simulink model "Quadrotor"  (R2017a)
settings: Solver=FixedStepAuto  StartTime=0.0  StopTime=12  FixedStep=0.001  RelTol=1e-3  EnableMultiTasking=on
values from neighbouring files (symbols this model uses):
  dU0 = 0*ones(Usize,1)    [go.m]
  U0 = 0*ones(Usize,1)    [go.m]
settings Model: Creator=stajeddi  LastModifiedBy=stajeddi
settings DataIOCC: LimitDataPoints=on
settings OptimizationCC: LifeSpan=inf
settings DebuggingCC: AllowSymbolicDim=off  SFUnexpectedBacktrackingDiag=warning  SFNoUnconditionalDefaultTransitionDiag=warning  SFExecutionAtInitializationDiag=none
settings ModelReferenceCC: PropagateSignalLabelsOutOfModel=off
settings GRTTargetCC: TargetLangStandard=C89/C90 (ANSI)
settings ConfigComp: CovMetricSettings=dw  CovHtmlReporting=on  CovSaveCumulativeToWorkspaceVar=on  CovSaveSingleToWorkspaceVar=on  CovExternalEMLEnable=off

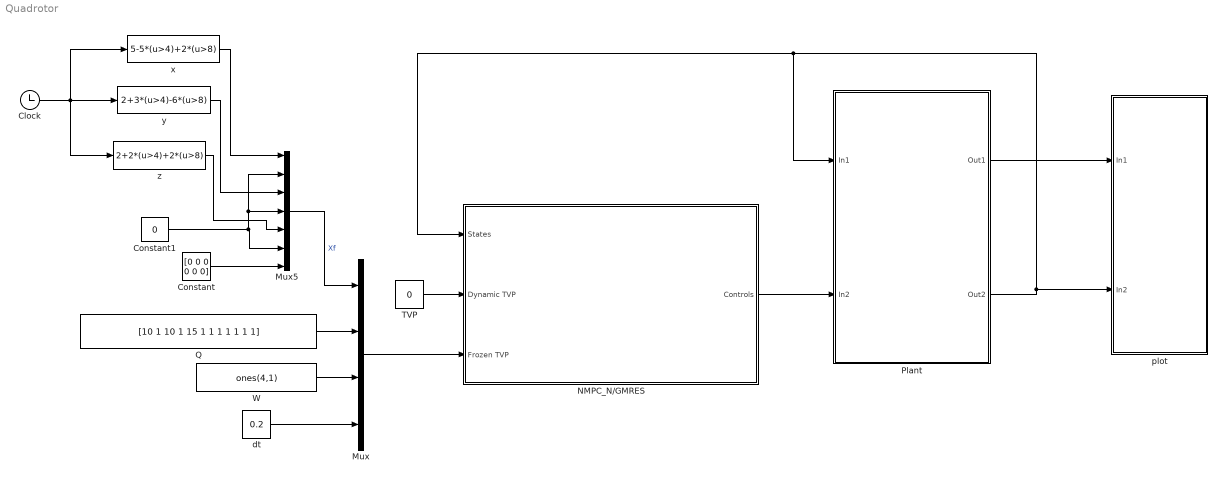
== system Quadrotor ==
  Clock : Clock
  Constant : Constant  Value=[0 0 0 0 0 0]
  Constant1 : Constant  Value=0
  Mux : Mux
  Mux5 : Mux  Inputs=7
  NMPC_N/GMRES : Subsystem
  Plant : Subsystem
  Q : Constant  Value=[10 1 10 1 15 1 1 1 1 1 1 1]
  TVP : Constant  Value=0
  W : Constant  Value=ones(4,1)
  dt : Constant  Value=0.2
  plot : Subsystem
  x : Fcn  Expr=5-5*(u>4)+2*(u>8)
  y : Fcn  Expr=2+3*(u>4)-6*(u>8)
  z : Fcn  Expr=2+2*(u>4)+2*(u>8)
  wires:
  Mux/1 -> NMPC_N/GMRES/3(Frozen TVP)
  Mux5/1 -> Mux/1  "Xf"
  Q/1 -> Mux/2
  W/1 -> Mux/3
  dt/1 -> Mux/4
  Constant/1 -> Mux5/7
  Constant1/1 -> Mux5/2, Mux5/4, Mux5/6
  Clock/1 -> y/1, x/1, z/1
  x/1 -> Mux5/1
  y/1 -> Mux5/3
  z/1 -> Mux5/5
  TVP/1 -> NMPC_N/GMRES/2(Dynamic TVP)
  Plant/2(Out2) -> Plant/1(In1), NMPC_N/GMRES/1(States), plot/2(In2)
  NMPC_N/GMRES/1(Controls) -> Plant/2(In2)
  Plant/1(Out1) -> plot/1(In1)

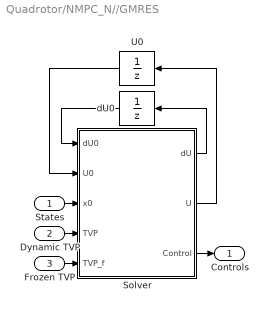
== system Quadrotor/NMPC_N//GMRES ==
  States : Inport
  Dynamic TVP : Inport  Port=2
  Frozen TVP : Inport  Port=3
  Solver : MATLAB Function  TreatAsAtomicUnit=on
  U0 : UnitDelay  InitialCondition=U0  SampleTime=-1
  dU0 : UnitDelay  InitialCondition=dU0  SampleTime=-1
  Controls : Outport
  wires:
  Dynamic TVP/1 -> Solver/4(TVP)
  dU0/1 -> Solver/1(dU0)
  Solver/1(dU) -> dU0/1
  U0/1 -> Solver/2(U0)
  Solver/2(U) -> U0/1
  Solver/3(Control) -> Controls/1
  Frozen TVP/1 -> Solver/5(TVP_f)
  States/1 -> Solver/3(x0)

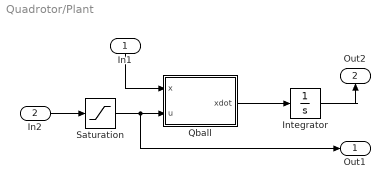
== system Quadrotor/Plant ==
  In1 : Inport
  In2 : Inport  Port=2
  Integrator : Integrator  InitialCondition=[0 0 0 0 0 0 0 0 0 0 0 0]'
  Qball : MATLAB Function  TreatAsAtomicUnit=on
  Saturation : Saturate  UpperLimit=inf  LowerLimit=0
  Out1 : Outport
  Out2 : Outport  Port=2
  wires:
  In1/1 -> Qball/1(x)
  Saturation/1 -> Out1/1, Qball/2(u)
  Integrator/1 -> Out2/1
  In2/1 -> Saturation/1
  Qball/1(xdot) -> Integrator/1

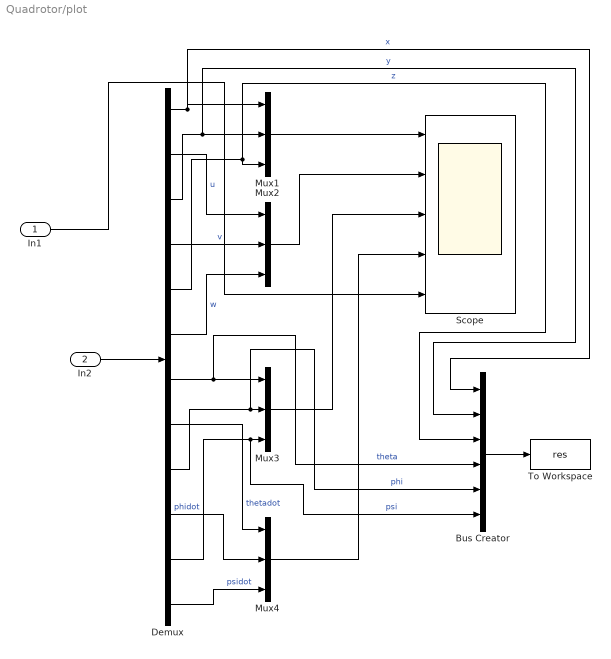
== system Quadrotor/plot ==
  In1 : Inport
  In2 : Inport  Port=2
  Bus Creator : BusCreator  Inputs=6
  Demux : Demux  Outputs=12
  Mux{1..4} (4 alike) : Mux  Inputs=3
  Scope : Scope  NumInputPorts=5
  To Workspace : ToWorkspace  VariableName=res  SaveFormat=Timeseries  SampleTime=-1
  wires:
  In1/1 -> Scope/5
  In2/1 -> Demux/1
  Demux/4 -> Mux2/2  "v"
  Demux/6 -> Mux2/3  "w"
  Demux/1 -> Mux1/1, Bus Creator/1  "x"
  Mux1/1 -> Scope/1
  Demux/3 -> Mux1/2, Bus Creator/2  "y"
  Demux/2 -> Mux2/1  "u"
  Demux/5 -> Bus Creator/3, Mux1/3  "z"
  Mux2/1 -> Scope/2
  Mux3/1 -> Scope/3
  Bus Creator/1 -> To Workspace/1
  Demux/10 -> Mux4/2  "phidot"
  Demux/7 -> Mux3/1, Bus Creator/4  "theta"
  Mux4/1 -> Scope/4
  Demux/8 -> Mux4/1  "thetadot"
  Demux/9 -> Bus Creator/5, Mux3/2  "phi"
  Demux/11 -> Bus Creator/6, Mux3/3  "psi"
  Demux/12 -> Mux4/3  "psidot"

== matlab function Quadrotor/NMPC_N//GMRES/Solver ==
  data: dU0 input; dU output; U0 input; x0 input; TVP input; U output; Control output; TVP_f input
%% NGMRES  NGMRES NGMRES
function [dU,U,Control] = NMPCBlock(dU0,U0,x0,TVP,TVP_f)
[dU,U,Control]=NMPC(dU0,U0,x0,TVP,TVP_f);

== matlab function Quadrotor/Plant/Qball ==
  data: x input; u input; xdot output
function xdot = Qball(x,u)
Xk1=x(1);
Xk2=x(2);
Xk3=x(3);
Xk4=x(4);
Xk5=x(5);
Xk6=x(6);
Xk7=x(7);
Xk8=x(8);
Xk9=x(9);
Xk10=x(10);
Xk11=x(11);
Xk12=x(12);
Uk1=u(1);
Uk2=u(2);
Uk3=u(3);
Uk4=u(4);
xdot=zeros(12,1);
xdot(1)=Xk2;
xdot(2)=(5*(sin(Xk9)*sin(Xk11) + cos(Xk9)*cos(Xk11)*sin(Xk7))*(Uk1 + Uk2 + Uk3 + Uk4))/7;
xdot(3)=Xk4;
xdot(4)=-(5*(cos(Xk11)*sin(Xk9) - cos(Xk9)*sin(Xk7)*sin(Xk11))*(Uk1 + Uk2 + Uk3 + Uk4))/7;
xdot(5)=Xk6;
xdot(6)=(5*cos(Xk7)*cos(Xk9)*(Uk1 + Uk2 + Uk3 + Uk4))/7 - 981/100;
xdot(7)=Xk8;
xdot(8)=(20*Uk1)/3 - (20*Uk2)/3;
xdot(9)=Xk10;
xdot(10)=(20*Uk3)/3 - (20*Uk4)/3;
xdot(11)=Xk12;
xdot(12)=100*Uk1 + 100*Uk2 - 100*Uk3 - 100*Uk4;
